simulink model "one_user"  (Simulink 8.1)
settings: Solver=FixedStepDiscrete  StartTime=0.0  StopTime=100  FixedStep=0.1  RelTol=1e-3
settings Model: Creator=hengyuj  LastModifiedBy=hengyuj
settings DataIOCC: SignalLoggingName=sigsOut
settings OptimizationCC: ExpressionDepthLimit=128
settings DebuggingCC: SaveWithParameterizedLinksMsg=none  SignalResolutionControl=TryResolveAllWithWarning  SolverPrmCheckMsg=none  MultiTaskDSMMsg=warning  MultiTaskCondExecSysMsg=none  FcnCallInpInsideContextMsg=EnableAllAsError  StrictBusMsg=None
settings HardwareCC: TargetUnknown=on
settings SFSimCC: SimParseCustomCode=off
settings RTWCC: IncludeERTFirstTime=on

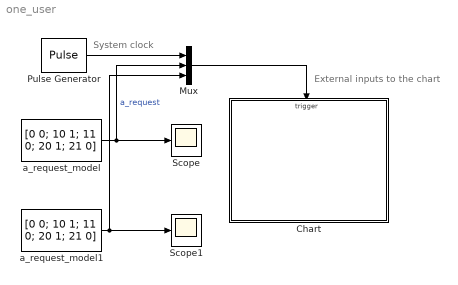
== system one_user ==
  note: System clock
  note: External inputs to the chart
  Chart : Stateflow chart  TreatAsAtomicUnit=on
  Mux : Mux  Inputs=3
  Pulse Generator : DiscretePulseGenerator  PulseType=Time based  Period=1  PulseWidth=50
  Scope : Scope
  Scope1 : Scope
  a_request_model : FromWorkspace  VariableName=[0 0; 10 1; 11 0; 20 1; 21 0]  SampleTime=0  Interpolate=off  OutputAfterFinalValue=Holding final value
  a_request_model1 : FromWorkspace  VariableName=[0 0; 10 1; 11 0; 20 1; 21 0]  SampleTime=0  Interpolate=off  OutputAfterFinalValue=Holding final value
  wires:
  a_request_model/1 -> Scope/1, Mux/2  "a_request"
  Mux/1 -> Chart/Trigger
  Pulse Generator/1 -> Mux/1
  a_request_model1/1 -> Scope1/1, Mux/3

== stateflow chart Chart ==
  note: 1- _0, _1, _2 refer to the states
      |     in the lecture notes.
      | 2- Run the simulation to see the
      |     execution of the current model.
      |     You can use Tools/Debug to
      |     enable/disable the animation.
      | 3- "a_request" event is an input
      |     from Simulink. You will need
      |     a second input for "user b".
  state Shared_Resource
    state a_USER [parallel]
      settings: executionOrder=1
      state idle_0
      state acquired_1
        en:
        tmp=t+1; /*ml.exprnd(1);*/
      state done_2
        tmp=t+ml.exprnd(10);
      (default) -> Shared_Resource.a_USER.idle_0
      Shared_Resource.a_USER.done_2 -> Shared_Resource.a_USER.idle_0 : [t>tmp]/release;
      Shared_Resource.a_USER.acquired_1 -> Shared_Resource.a_USER.done_2 : [t>tmp]
      Shared_Resource.a_USER.idle_0 -> (junction 16) : a_request
      (junction 16) -> Shared_Resource.a_USER.idle_0 [order 1] : [r_in_use==1]
      (junction 16) -> Shared_Resource.a_USER.acquired_1 [order 2] : [r_in_use==0]/acquire;
    state Resource [parallel]
      settings: executionOrder=2
      state idle_0
        en: r_in_use=0;
      state busy_2
        en:
        r_in_use=1;
      busy_2 -> Shared_Resource.Resource.idle_0 : release
      Shared_Resource.Resource.idle_0 -> busy_2 : acquire
    state b_USER [parallel]
      settings: executionOrder=3
      state idle_0
      state acquired_1
        en:
        tmp=t+1; /*ml.exprnd(1);*/
      state done_2
        tmp=t+ml.exprnd(10);
      (default) -> Shared_Resource.b_USER.idle_0
      Shared_Resource.b_USER.done_2 -> Shared_Resource.b_USER.idle_0 : [t>tmp]/release;
      Shared_Resource.b_USER.acquired_1 -> Shared_Resource.b_USER.done_2 : [t>tmp]
      Shared_Resource.b_USER.idle_0 -> (junction 26) : b_request
      (junction 26) -> Shared_Resource.b_USER.idle_0 [order 1] : [r_in_use==1]
      (junction 26) -> Shared_Resource.b_USER.acquired_1 [order 2] : [r_in_use==0]/acquire;
    (default) -> Shared_Resource.Resource.idle_0
  data: r_in_use local double; tmp local double
  events: acquire local EITHER_EDGE_EVENT; release local EITHER_EDGE_EVENT; use local EITHER_EDGE_EVENT; clock input RISING_EDGE_EVENT; a_request input RISING_EDGE_EVENT; b_request input RISING_EDGE_EVENT
